simulink model "Gray_Processing"  (R2013b)
settings: Solver=ode45  StartTime=0.0  StopTime=1000  RelTol=1e-3
InitFcn:
  | %% DSPBuilder Start
  | alt_dspbuilder_update_model(bdroot)
  | %% DSPBuilder End
libraries: allblocks_alteradspbuilder2 x23, simulink x3
settings Model: Creator=Given_Jiang  LastModifiedBy=Given_Jiang

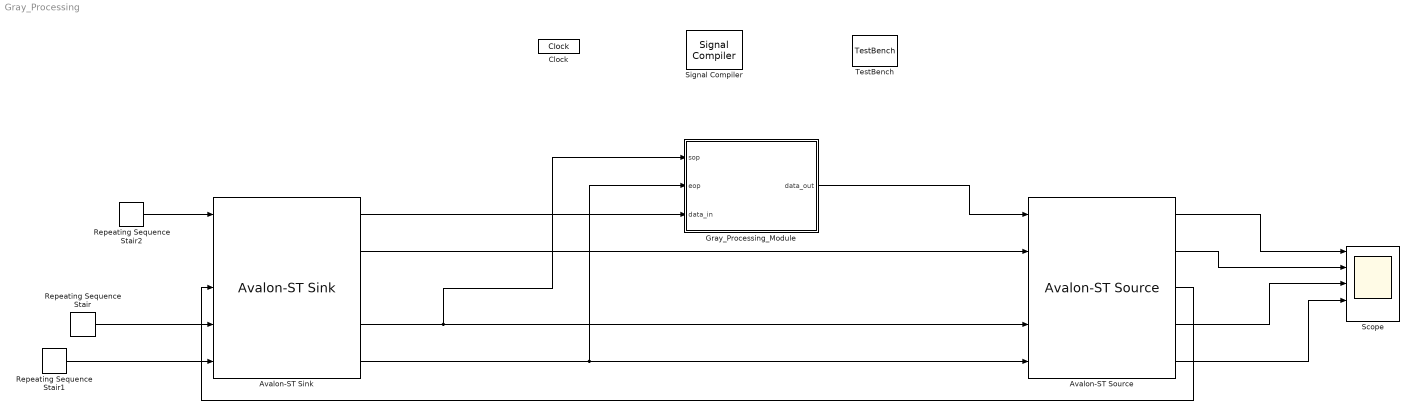
== system Gray_Processing ==
  Avalon-ST Sink : allblocks_alteradspbuilder2/Avalon-ST Sink  iofile=E:\FPGA\SOC\Quartus\quartus\dsp_builder\design\VIP_LIB\Gray_Processing\tb_Gray_Processing\Gray%5FProcessing_Avalon-ST+Sink_data.salt,E:\FPGA\SOC\Quartus\quartus\dsp_builder\design\VIP_LIB\Gray_Processing\tb_Gray_Processing\Gray%5FProcessing_Avalon-ST+Sink_valid.salt,E:\FPGA\SOC\Quartus\quartus\dsp_builder\design\VIP_LIB\Gray_Processing\tb_Gray_Processing\Gray%5FProcessing_Avalon-ST+Sink_ready.capture,E:\FPGA\SOC\Quartus\quartus\dsp_builder\design\VIP_LIB\Gray_Processing\tb_Gray_Processing\Gray%5FProcessing_Avalon-ST+Sink_startofpacket.salt,E:\FPGA\SOC\Quartus\quartus\dsp_builder\design\VIP_LIB\Gray_Processing\tb_Gray_Processing\Gray%5FProcessing_Avalon-ST+Sink_endofpacket.salt,  SpecifyClock=off  BusType=Unsigned Integer  bwl=24  bwr=0  symbolWidth=8  symbolsPerBeat=3  numOfChannels=0  numOfErrorDescriptors=0  endOfPacket=on  startOfPacket=on  empty=off  readyLatency=1  externalType=Inferred  PORTTYPE=Output
  Avalon-ST Source : allblocks_alteradspbuilder2/Avalon-ST Source  iofile=E:\FPGA\SOC\Quartus\quartus\dsp_builder\design\VIP_LIB\Gray_Processing\tb_Gray_Processing\Gray%5FProcessing_Avalon-ST+Source_data.capture,E:\FPGA\SOC\Quartus\quartus\dsp_builder\design\VIP_LIB\Gray_Processing\tb_Gray_Processing\Gray%5FProcessing_Avalon-ST+Source_valid.capture,E:\FPGA\SOC\Quartus\quartus\dsp_builder\design\VIP_LIB\Gray_Processing\tb_Gray_Processing\Gray%5FProcessing_Avalon-ST+Source_ready.salt,E:\FPGA\SOC\Quartus\quartus\dsp_builder\design\VIP_LIB\Gray_Processing\tb_Gray_Processing\Gray%5FProcessing_Avalon-ST+Source_startofpacket.capture,E:\FPGA\SOC\Quartus\quartus\dsp_builder\design\VIP_LIB\Gray_Processing\tb_Gray_Processing\Gray%5FProcessing_Avalon-ST+Source_endofpacket.capture,  SpecifyClock=off  BusType=Unsigned Integer  bwl=24  bwr=0  symbolWidth=8  symbolsPerBeat=3  numOfChannels=0  numOfErrorDescriptors=0  endOfPacket=on  startOfPacket=on  empty=off  readyLatency=1  externalType=Inferred  PORTTYPE=Input
  Clock : allblocks_alteradspbuilder2/Clock  ClockPeriod=7.5  ClockPeriodUnit=ns  SampleTime=1  ResetLatency=0  ResetRegisterCascadeDepth=0  SimulationStartCycle=5  PhaseOffset=0  Reset=aclr  ResetType=Active Low  Export=off
  Gray_Processing_Module : Subsystem
  Repeating Sequence Stair : simulink/Sources/Repeating Sequence Stair  OutValues=[1 0 0 0 1 0 0 0 0 0].'  tsamp=-1  OutMin=[]  OutMax=[]  OutDataTypeStr=double  OutputDataTypeScalingMode=double  OutDataType=fixdt(0,8)  ConRadixGroup=Best Precision: Vector-wise  OutScaling=2^-12
  Repeating Sequence Stair1 : simulink/Sources/Repeating Sequence Stair  OutValues=[0 0 0 1 0 0 0 0 0 1].'  tsamp=-1  OutMin=[]  OutMax=[]  OutDataTypeStr=double  OutputDataTypeScalingMode=double  OutDataType=fixdt(0,8)  ConRadixGroup=Best Precision: Vector-wise  OutScaling=2^-12
  Repeating Sequence Stair2 : simulink/Sources/Repeating Sequence Stair  OutValues=[15 101 102 103 0 65793 66305 189 190 254].'  tsamp=-1  OutMin=[]  OutMax=[]  OutDataTypeStr=double  OutputDataTypeScalingMode=double  OutDataType=fixdt(0,8)  ConRadixGroup=Best Precision: Vector-wise  OutScaling=2^-12
  Scope : Scope  NumInputPorts=5
      settings: YMin=-5~-5~-5~-5~-5  YMax=5~5~5~5~5
  Signal Compiler : allblocks_alteradspbuilder2/Signal Compiler  DeviceFamily=Cyclone V  DeviceName=AUTO  DisableEarlyHDLGeneration=off  EnableSignalTap=off  SignalTapDepth=128  UseBoardBlock=off  StpUseDefaultClock=on  StpClock=Clock  ExportDir=E:\FPGA\SOC\Quartus\quartus\dsp_builder
  TestBench : allblocks_alteradspbuilder2/TestBench  enable=on  advancedMode=on  modelSimGui=off  maxDisplayErrors=10  mismatchErrorLevel=Error  simdatafile=E:\FPGA\SOC\Quartus\quartus\dsp_builder\design\VIP_LIB\Gray_Processing\tb_Gray_Processing\Gray_Processing.simdata.tcl
  wires:
  Avalon-ST Sink/2 -> Avalon-ST Source/2
  Avalon-ST Source/3 -> Avalon-ST Sink/3
  Avalon-ST Sink/4 -> Gray_Processing_Module/1(sop), Avalon-ST Source/4
  Avalon-ST Sink/5 -> Gray_Processing_Module/2(eop), Avalon-ST Source/5
  Avalon-ST Sink/1 -> Gray_Processing_Module/3(data_in)
  Gray_Processing_Module/1(data_out) -> Avalon-ST Source/1
  Repeating Sequence Stair/1 -> Avalon-ST Sink/4
  Repeating Sequence Stair1/1 -> Avalon-ST Sink/5
  Repeating Sequence Stair2/1 -> Avalon-ST Sink/1
  Avalon-ST Source/1 -> Scope/1
  Avalon-ST Source/2 -> Scope/2
  Avalon-ST Source/4 -> Scope/3
  Avalon-ST Source/5 -> Scope/4

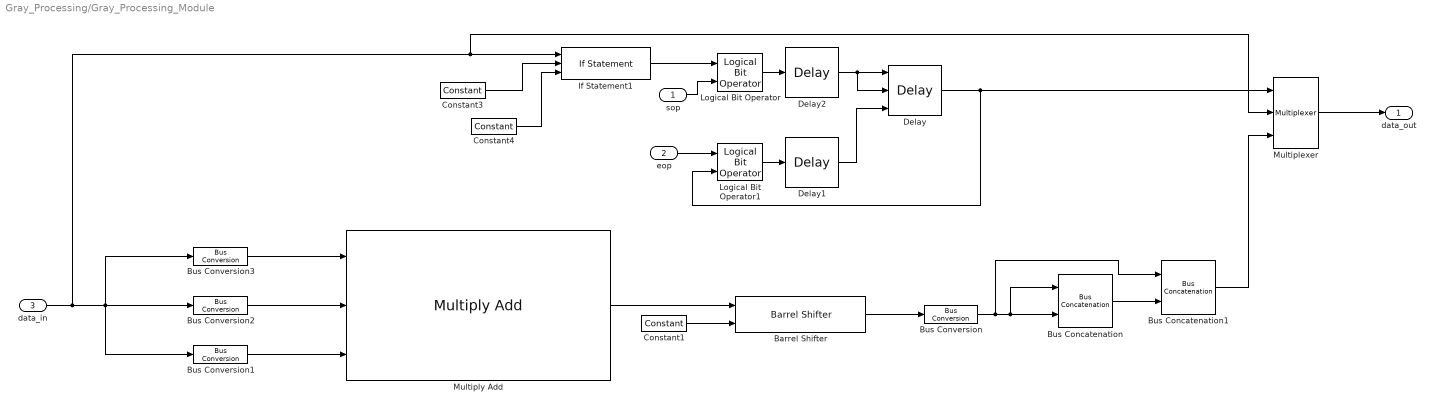
== system Gray_Processing/Gray_Processing_Module ==
  sop : Inport
  eop : Inport  Port=2
  data_in : Inport  Port=3
  Barrel Shifter : allblocks_alteradspbuilder2/Barrel Shifter  BusType=Unsigned Integer  bwl=18  bwr=8  pipeline=off  infer_distance=off  distance_length=4  ShiftDirection=Shift right  use_ena=off  use_aclr=off  UseDedicatedCircuitry=off  pipeline_display=0  allowFloatingPointOverride=on  logOutputs=off  logFile=E:\FPGA\SOC\Quartus\quartus\dsp_builder\design\VIP_LIB\Gray_Processing\tb_Gray_Processing\Gray%5FProcessing_Gray%5FProcessing%5FModule_Barrel+Shifter.fixedpointlog
  Bus Concatenation : allblocks_alteradspbuilder2/Bus Concatenation  isSigned=off  awidth=8  bwidth=8  pipeline_display=0
  Bus Concatenation1 : allblocks_alteradspbuilder2/Bus Concatenation  isSigned=off  awidth=8  bwidth=16  pipeline_display=0
  Bus Conversion : allblocks_alteradspbuilder2/Bus Conversion  BusType=Unsigned Integer  ibwl=18  ibwr=1  bwl=8  bwr=1  bitToConnectToOutputLSB=0  round=off  saturate=off  pipeline_display=0
  Bus Conversion1 : allblocks_alteradspbuilder2/Bus Conversion  BusType=Unsigned Integer  ibwl=24  ibwr=1  bwl=8  bwr=1  bitToConnectToOutputLSB=0  round=off  saturate=off  pipeline_display=0
  Bus Conversion2 : allblocks_alteradspbuilder2/Bus Conversion  BusType=Unsigned Integer  ibwl=24  ibwr=1  bwl=8  bwr=1  bitToConnectToOutputLSB=8  round=off  saturate=off  pipeline_display=0
  Bus Conversion3 : allblocks_alteradspbuilder2/Bus Conversion  BusType=Unsigned Integer  ibwl=24  ibwr=1  bwl=8  bwr=1  bitToConnectToOutputLSB=16  round=off  saturate=off  pipeline_display=0
  Constant1 : allblocks_alteradspbuilder2/Constant  mask_cst=8  BusType=Unsigned Integer  bwl=4  bwr=0  roundMode=Truncate  satMode=Wrap  SpecifyClock=off  allowFloatingPointOverride=on  logOutputs=off  logFile=E:\FPGA\SOC\Quartus\quartus\dsp_builder\design\VIP_LIB\Gray_Processing\tb_Gray_Processing\Gray%5FProcessing_Gray%5FProcessing%5FModule_Constant1.fixedpointlog
  Constant3 : allblocks_alteradspbuilder2/Constant  mask_cst=0  BusType=Unsigned Integer  bwl=24  bwr=0  roundMode=Truncate  satMode=Wrap  SpecifyClock=off  allowFloatingPointOverride=on  logOutputs=off  logFile=E:\FPGA\SOC\Quartus\quartus\dsp_builder\design\VIP_LIB\Gray_Processing\tb_Gray_Processing\Gray%5FProcessing_Gray%5FProcessing%5FModule_Constant3.fixedpointlog
  Constant4 : allblocks_alteradspbuilder2/Constant  mask_cst=15  BusType=Unsigned Integer  bwl=24  bwr=0  roundMode=Truncate  satMode=Wrap  SpecifyClock=off  allowFloatingPointOverride=on  logOutputs=off  logFile=E:\FPGA\SOC\Quartus\quartus\dsp_builder\design\VIP_LIB\Gray_Processing\tb_Gray_Processing\Gray%5FProcessing_Gray%5FProcessing%5FModule_Constant4.fixedpointlog
  Delay : allblocks_alteradspbuilder2/Delay  pipeline=1  pipeline_display=1  ClockPhase=1  use_ena=on  use_sclr=on  allowFloatingPointOverride=on  logOutputs=off  logFile=E:\FPGA\SOC\Quartus\quartus\dsp_builder\design\VIP_LIB\Gray_Processing\tb_Gray_Processing\Gray%5FProcessing_Gray%5FProcessing%5FModule_Delay.fixedpointlog  use_init=on  reset_value=0
  Delay1 : allblocks_alteradspbuilder2/Delay  pipeline=1  pipeline_display=1  ClockPhase=1  use_ena=off  use_sclr=off  allowFloatingPointOverride=on  logOutputs=off  logFile=E:\FPGA\SOC\Quartus\quartus\dsp_builder\design\VIP_LIB\Gray_Processing\tb_Gray_Processing\Gray%5FProcessing_Gray%5FProcessing%5FModule_Delay1.fixedpointlog  use_init=off  reset_value=0
  Delay2 : allblocks_alteradspbuilder2/Delay  pipeline=1  pipeline_display=1  ClockPhase=1  use_ena=off  use_sclr=off  allowFloatingPointOverride=on  logOutputs=off  logFile=E:\FPGA\SOC\Quartus\quartus\dsp_builder\design\VIP_LIB\Gray_Processing\tb_Gray_Processing\Gray%5FProcessing_Gray%5FProcessing%5FModule_Delay2.fixedpointlog  use_init=off  reset_value=0
  If Statement1 : allblocks_alteradspbuilder2/If Statement  user_inputs=3  if_expression=(a=b)&(a~c)  BusType=Unsigned Integer  bwl=24  bwr=0  pipeline_display=1  use_else_output=off  use_elseif_input=off
  Logical Bit Operator : allblocks_alteradspbuilder2/Logical Bit Operator  LogicalOperator=AND  user_inputs=2  pipeline_display=0
  Logical Bit Operator1 : allblocks_alteradspbuilder2/Logical Bit Operator  LogicalOperator=AND  user_inputs=2  pipeline_display=0
  Multiplexer : allblocks_alteradspbuilder2/Multiplexer  numInputs=2  pipeline=0  oneHot=off  pipeline_display=0  use_ena=off  use_aclr=off  allowFloatingPointOverride=on  logOutputs=off  logFile=E:\FPGA\SOC\Quartus\quartus\dsp_builder\design\VIP_LIB\Gray_Processing\tb_Gray_Processing\Gray%5FProcessing_Gray%5FProcessing%5FModule_Multiplexer.fixedpointlog
  Multiply Add : allblocks_alteradspbuilder2/Multiply Add  multipliers=3  BusType=Unsigned Integer  bwl=8  bwr=0  direction=Add Add  pipeline_register=No Register  pipeline_display=0  use_constants=on  constants=[76 150 30]  UseDedicatedCircuitry=on  use_ena=off  use_aclr=off  allowFloatingPointOverride=on  logOutputs=off  logFile=E:\FPGA\SOC\Quartus\quartus\dsp_builder\design\VIP_LIB\Gray_Processing\tb_Gray_Processing\Gray%5FProcessing_Gray%5FProcessing%5FModule_Multiply+Add.fixedpointlog
  data_out : Outport
  wires:
  If Statement1/1 -> Logical Bit Operator/1
  Delay/1 -> Logical Bit Operator1/2, Multiplexer/1
  sop/1 -> Logical Bit Operator/2
  data_in/1 -> If Statement1/1, Multiplexer/2, Bus Conversion1/1, Bus Conversion2/1, Bus Conversion3/1
  Multiplexer/1 -> data_out/1
  Constant3/1 -> If Statement1/2
  Constant4/1 -> If Statement1/3
  eop/1 -> Logical Bit Operator1/1
  Logical Bit Operator1/1 -> Delay1/1
  Delay1/1 -> Delay/3
  Barrel Shifter/1 -> Bus Conversion/1
  Bus Conversion/1 -> Bus Concatenation1/1, Bus Concatenation/1, Bus Concatenation/2
  Bus Concatenation/1 -> Bus Concatenation1/2
  Bus Concatenation1/1 -> Multiplexer/3
  Constant1/1 -> Barrel Shifter/2
  Bus Conversion3/1 -> Multiply Add/1
  Bus Conversion2/1 -> Multiply Add/2
  Bus Conversion1/1 -> Multiply Add/3
  Logical Bit Operator/1 -> Delay2/1
  Delay2/1 -> Delay/2, Delay/1
  Multiply Add/1 -> Barrel Shifter/1
